simulink model "ES249B_MotAgCorrln"  (R2013b)
settings: Solver=FixedStepDiscrete  SolverMode=SingleTasking  StartTime=0.0  StopTime=1  FixedStep=0.002  RelTol=1e-3
values from neighbouring files (symbols this model uses):
  FLTINJ_MOTAGCORRLN_MOTAGIDPTSIG = DataDict.Constant    [ES249B_MotAgCorrln_DataDict.m]
  HALFREV_MOTREV_U0P16 = DataDict.Constant    [ES249B_MotAgCorrln_DataDict.m]
  MOTAGACORRLNST_CNT_U08 = DataDict.Constant    [ES249B_MotAgCorrln_DataDict.m]
  MotAgAMotAgBCorrln = DataDict.NTC    [ES249B_MotAgCorrln_DataDict.m]
  MOTAGBCORRLNST_CNT_U08 = DataDict.Constant    [ES249B_MotAgCorrln_DataDict.m]
  MOTAGCORRLNERRTHD_MOTREVELEC_U0P16 = DataDict.Constant    [ES249B_MotAgCorrln_DataDict.m]
  MOTAGCORRLNNTCFAILSTEP_CNT_U16 = DataDict.Constant    [ES249B_MotAgCorrln_DataDict.m]
  MOTAGCORRLNNTCPASSSTEP_CNT_U16 = DataDict.Constant    [ES249B_MotAgCorrln_DataDict.m]
  MOTAGMAXSTALLCNTR_CNT_U08 = DataDict.Constant    [ES249B_MotAgCorrln_DataDict.m]
  MotAgMeclCorrlnSt = DataDict.OpSignal    [ES249B_MotAgCorrln_DataDict.m]
  MotAgMeclIdptSig = DataDict.OpSignal    [ES249B_MotAgCorrln_DataDict.m]
  SysGlbPrmMotPoleCnt = DataDict.ImprtdCal    [ES249B_MotAgCorrln_DataDict.m]
undefined symbols (not defined in the file or in its folder): NtcSts1, sigbuilder_block, SigQlfr1
libraries: simulink x5
(part 2 of 2)

== system ES249B_MotAgCorrln/MotAgCorrln/MotAgCorrlnPer1/MtrAgB SigAvlCheck ==
  note: Example of PIM declaration for StallCnt State Variable
      |
      | SnsrShoNameSens0StallCntPrev = DataDict.PIM;
      | SnsrShoNameSens0StallCntPrev.LongName = 'SnsrShoNameSens0RollgCntPrev';
      | SnsrShoNameSens0StallCntPrev.Description = 'SnsrShoNameSens0RollgCntPrev';
      | SnsrShoNameSens0StallCntPrev.DocUnits = 'Cnt';
      | SnsrShoNameSens0StallCntPrev.EngDT = dt.u08;
      | SnsrShoNameSens0StallCntPrev.EngInit = 0;
      | SnsrShoNameSens0StallCntPrev.EngMin = 0;
      | SnsrShoNameSens0StallCntPrev.EngMax = 255;
      |
      |
      | *********  Need different state variable for each instance of this  subsystem ********
  note: Example of PIM declaration for RollgCnt State Variable
      |
      | SnsrShoNameSens0RollgCntPrev = DataDict.PIM;
      | SnsrShoNameSens0RollgCntPrev.LongName = 'SnsrShoNameSens0RollgCntPrev';
      | SnsrShoNameSens0RollgCntPrev.Description = 'SnsrShoNameSens0RollgCntPrev';
      | SnsrShoNameSens0RollgCntPrev.DocUnits = 'Cnt';
      | SnsrShoNameSens0RollgCntPrev.EngDT = dt.u08;
      | SnsrShoNameSens0RollgCntPrev.EngInit = 0;
      | SnsrShoNameSens0RollgCntPrev.EngMin = 0;
      | SnsrShoNameSens0RollgCntPrev.EngMax = 255;
      |
      |
      | *********  Need different state variable for each instance of this  subsystem ********
  SigRollgCnt : Inport  OutDataTypeStr=uint8
  SigQlfr : Inport  Port=2  OutDataTypeStr=uint8
  kMaxStallCnt : Inport  Port=3  OutDataTypeStr=uint8
  Copyright1 : Subsystem  Description=|  RequirementInfo={} %GIDa_9de21268_1023_46e5_9fbe_013ff02661ff  mask(Copyright Information){none=on}
      | Copyright info block.                                               
      |                                                                     
      | Place copyright information at the top of every subsystem in design.
      mask prompts: none "No parameters"
      mask help: Place copyright information at the top of every subsystem in design.
      mask Display:
      | NxtrConf = 'Nexteer Confidential';
      | 
      | sys = bdroot; %handle for the current model ("system")
      | first = get_param(sys,'Created');
      | if(isempty(first))
      |     first = datestr(now,'yyyy');
      | else
      |     first = first(end-3:end);  %year is last four digits
      | end
      | 
      | last = get_param(sys,'LastModifiedDate');
      | if isempty(last)
      |     last = datestr(now,'yyyy');
      | else
      |     last = last(end-3:end);
      | end
      | 
      | if strcmp(first,last)
      |     fprintf('%s\nCopyright  %s Nexteer',NxtrConf,first);
      | else
      |     fprintf('%s\n%s%s-%s Nexteer',NxtrConf,char(169),first,last);
      | end
  CorrSigAvlChkRev1 : Stateflow chart  TreatAsAtomicUnit=on
  Unit Delay : UnitDelay  SampleTime=-1  StateName=MotAgCorrlnMotAgBRollgCntPrev  StateMustResolveToSignalObject=on
      settings: AttributesFormatString=|
      | State Variable:
      | %<StateName>
  Unit Delay1 : UnitDelay  SampleTime=-1  StateName=MotAgCorrlnMotAgBStallCntPrev  StateMustResolveToSignalObject=on
      settings: AttributesFormatString=|
      | State Variable:
      | %<StateName>
  SigAvl : Outport
  wires:
  SigRollgCnt/1 -> Unit Delay/1, CorrSigAvlChkRev1/1(SigRollgCnt)  "SigRollgCnt"
  SigQlfr/1 -> CorrSigAvlChkRev1/2(SigQlfr)  "SigQlfr"
  kMaxStallCnt/1 -> CorrSigAvlChkRev1/3(kMaxStallCnt)  "kMaxStallCnt"
  Unit Delay/1 -> CorrSigAvlChkRev1/4(LstRollgCnt)
  CorrSigAvlChkRev1/2(StallCntOutp) -> Unit Delay1/1
  Unit Delay1/1 -> CorrSigAvlChkRev1/5(LstStallCnt)
  CorrSigAvlChkRev1/1(SigAvl) -> SigAvl/1

== system ES249B_MotAgCorrln/MotAgCorrln/MotAgCorrlnInit1/Compute Error Threshold/Copyright1 ==

== system ES249B_MotAgCorrln/MotAgCorrln/MotAgCorrlnPer1/Build Correlation Status/Copyright1 ==

== system ES249B_MotAgCorrln/MotAgCorrln/MotAgCorrlnPer1/DetermineIndSignals/Fail Action  ==
  Action Port : ActionPort  ActionType=else
  Constant : Constant  Value=0  OutDataTypeStr=uint8
      settings: AttributesFormatString=%<OutDataTypeStr>
  Copyright1 : Subsystem  Description=|  mask(Copyright Information){none=on}
      | Copyright info block.                                               
      |                                                                     
      | Place copyright information at the top of every subsystem in design.
      mask prompts: none "No parameters"
      mask help: Place copyright information at the top of every subsystem in design.
      mask Display:
      | NxtrConf = 'Nexteer Confidential';
      | 
      | sys = bdroot; %handle for the current model ("system")
      | first = get_param(sys,'Created');
      | if(isempty(first))
      |     first = datestr(now,'yyyy');
      | else
      |     first = first(end-3:end);  %year is last four digits
      | end
      | 
      | last = get_param(sys,'LastModifiedDate');
      | if isempty(last)
      |     last = datestr(now,'yyyy');
      | else
      |     last = last(end-3:end);
      | end
      | 
      | if strcmp(first,last)
      |     fprintf('%s\nCopyright  %s Nexteer',NxtrConf,first);
      | else
      |     fprintf('%s\n%s%s-%s Nexteer',NxtrConf,char(169),first,last);
      | end
  MotAgMeclIdptSig : Outport  OutDataTypeStr=uint8
  wires:
  Constant/1 -> MotAgMeclIdptSig/1

== system ES249B_MotAgCorrln/MotAgCorrln/MotAgCorrlnPer1/DetermineIndSignals/Pass Action  ==
  Action Port : ActionPort  ActionType=then
  Constant : Constant  Value=MotAgMeclIdptSig.EngMax  OutDataTypeStr=uint8
      settings: AttributesFormatString=%<OutDataTypeStr>
  Copyright1 : Subsystem  Description=|  mask(Copyright Information){none=on}
      | Copyright info block.                                               
      |                                                                     
      | Place copyright information at the top of every subsystem in design.
      mask prompts: none "No parameters"
      mask help: Place copyright information at the top of every subsystem in design.
      mask Display:
      | NxtrConf = 'Nexteer Confidential';
      | 
      | sys = bdroot; %handle for the current model ("system")
      | first = get_param(sys,'Created');
      | if(isempty(first))
      |     first = datestr(now,'yyyy');
      | else
      |     first = first(end-3:end);  %year is last four digits
      | end
      | 
      | last = get_param(sys,'LastModifiedDate');
      | if isempty(last)
      |     last = datestr(now,'yyyy');
      | else
      |     last = last(end-3:end);
      | end
      | 
      | if strcmp(first,last)
      |     fprintf('%s\nCopyright  %s Nexteer',NxtrConf,first);
      | else
      |     fprintf('%s\n%s%s-%s Nexteer',NxtrConf,char(169),first,last);
      | end
  MotAgMeclIdptSig : Outport
  wires:
  Constant/1 -> MotAgMeclIdptSig/1

== system ES249B_MotAgCorrln/MotAgCorrln/MotAgCorrlnPer1/FltInj_u08 /Copyright1 ==

== system ES249B_MotAgCorrln/MotAgCorrln/MotAgCorrlnPer1/GetNtcQlfrSts 0x080 /CopyRight2 ==

== system ES249B_MotAgCorrln/MotAgCorrln/MotAgCorrlnPer1/MotAgA vs MotAgB/Copyright1 ==

== system ES249B_MotAgCorrln/MotAgCorrln/MotAgCorrlnPer1/MotAgA vs MotAgB/Fails the test ==
  Action Port : ActionPort  ActionType=else
  Copyright1 : Subsystem  Description=|  mask(Copyright Information){none=on}
      | Copyright info block.                                               
      |                                                                     
      | Place copyright information at the top of every subsystem in design.
      mask prompts: none "No parameters"
      mask help: Place copyright information at the top of every subsystem in design.
      mask Display:
      | NxtrConf = 'Nexteer Confidential';
      | 
      | sys = bdroot; %handle for the current model ("system")
      | first = get_param(sys,'Created');
      | if(isempty(first))
      |     first = datestr(now,'yyyy');
      | else
      |     first = first(end-3:end);  %year is last four digits
      | end
      | 
      | last = get_param(sys,'LastModifiedDate');
      | if isempty(last)
      |     last = datestr(now,'yyyy');
      | else
      |     last = last(end-3:end);
      | end
      | 
      | if strcmp(first,last)
      |     fprintf('%s\nCopyright  %s Nexteer',NxtrConf,first);
      | else
      |     fprintf('%s\n%s%s-%s Nexteer',NxtrConf,char(169),first,last);
      | end
  MOTAGCORRLNNTCFAILSTEP_CNT_U16 : Constant  Value=MOTAGCORRLNNTCFAILSTEP_CNT_U16
  Parameter Byte : Constant  OutDataTypeStr=uint8
  Status Type : Constant  Value=NtcSts1.NTCSTS_PREFAILD
  NtcInfo : Outport  InitialOutput=1
  NtcSts : Outport  Port=2  InitialOutput=NtcSts1.NTCSTS_PREFAILD
  DebStep : Outport  Port=3  InitialOutput=MOTAGCORRLNNTCFAILSTEP_CNT_U16
  wires:
  MOTAGCORRLNNTCFAILSTEP_CNT_U16/1 -> DebStep/1
  Status Type/1 -> NtcSts/1
  Parameter Byte/1 -> NtcInfo/1

== system ES249B_MotAgCorrln/MotAgCorrln/MotAgCorrlnPer1/MotAgA vs MotAgB/Passes the test ==
  Action Port : ActionPort  ActionType=then
  Copyright1 : Subsystem  Description=|  mask(Copyright Information){none=on}
      | Copyright info block.                                               
      |                                                                     
      | Place copyright information at the top of every subsystem in design.
      mask prompts: none "No parameters"
      mask help: Place copyright information at the top of every subsystem in design.
      mask Display:
      | NxtrConf = 'Nexteer Confidential';
      | 
      | sys = bdroot; %handle for the current model ("system")
      | first = get_param(sys,'Created');
      | if(isempty(first))
      |     first = datestr(now,'yyyy');
      | else
      |     first = first(end-3:end);  %year is last four digits
      | end
      | 
      | last = get_param(sys,'LastModifiedDate');
      | if isempty(last)
      |     last = datestr(now,'yyyy');
      | else
      |     last = last(end-3:end);
      | end
      | 
      | if strcmp(first,last)
      |     fprintf('%s\nCopyright  %s Nexteer',NxtrConf,first);
      | else
      |     fprintf('%s\n%s%s-%s Nexteer',NxtrConf,char(169),first,last);
      | end
  MOTAGCORRLNNTCPASSSTEP_CNT_U16 : Constant  Value=MOTAGCORRLNNTCPASSSTEP_CNT_U16
  Parameter Byte Data1 : Constant  Value=0  OutDataTypeStr=uint8
  Status Type : Constant  Value=NtcSts1.NTCSTS_PREPASSD
  NtcInfo : Outport  InitialOutput=0
  NtcSts : Outport  Port=2  InitialOutput=NtcSts1.NTCSTS_PREPASSD
  DebStep : Outport  Port=3  InitialOutput=MOTAGCORRLNNTCPASSSTEP_CNT_U16
  wires:
  MOTAGCORRLNNTCPASSSTEP_CNT_U16/1 -> DebStep/1
  Status Type/1 -> NtcSts/1
  Parameter Byte Data1/1 -> NtcInfo/1

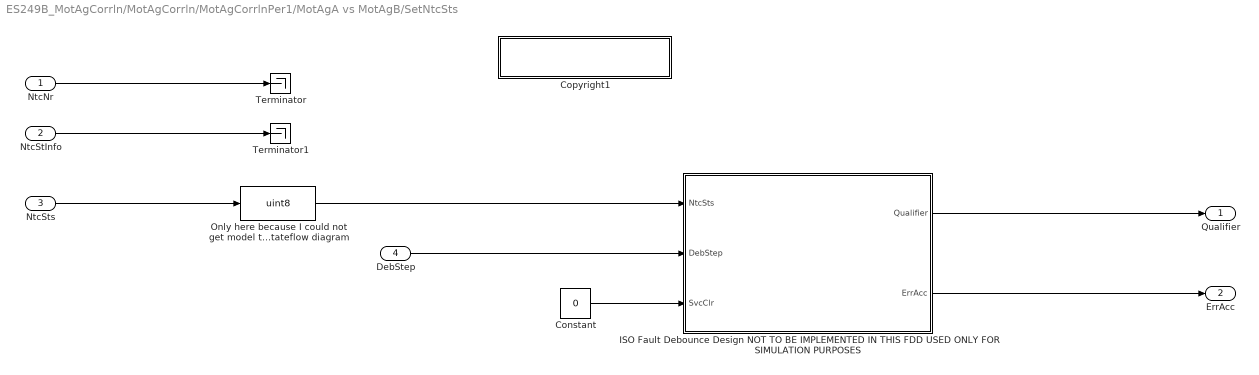
== system ES249B_MotAgCorrln/MotAgCorrln/MotAgCorrlnPer1/MotAgA vs MotAgB/SetNtcSts ==
  NtcNr : Inport
  NtcStInfo : Inport  Port=2
  NtcSts : Inport  Port=3  OutDataTypeStr=Enum: NtcSts1
  DebStep : Inport  Port=4  OutDataTypeStr=uint16
  Constant : Constant  Value=0
  Copyright1 : Subsystem  Description=|  mask(Copyright Information){none=on}
      | Copyright info block.                                               
      |                                                                     
      | Place copyright information at the top of every subsystem in design.
      mask prompts: none "No parameters"
      mask help: Place copyright information at the top of every subsystem in design.
      mask Display:
      | NxtrConf = 'Nexteer Confidential';
      | 
      | sys = bdroot; %handle for the current model ("system")
      | first = get_param(sys,'Created');
      | if(isempty(first))
      |     first = datestr(now,'yyyy');
      | else
      |     first = first(end-3:end);  %year is last four digits
      | end
      | 
      | last = get_param(sys,'LastModifiedDate');
      | if isempty(last)
      |     last = datestr(now,'yyyy');
      | else
      |     last = last(end-3:end);
      | end
      | 
      | if strcmp(first,last)
      |     fprintf('%s\nCopyright  %s Nexteer',NxtrConf,first);
      | else
      |     fprintf('%s\n%s%s-%s Nexteer',NxtrConf,char(169),first,last);
      | end
  ISO Fault Debounce Design NOT TO BE IMPLEMENTED IN THIS FDD USED ONLY FOR SIMULATION PURPOSES : Stateflow chart  TreatAsAtomicUnit=on
  Only here because I could not get model to run with enumerations in the stateflow diagram : DataTypeConversion  OutDataTypeStr=uint8
  Terminator : Terminator
  Terminator1 : Terminator
  Qualifier : Outport
  ErrAcc : Outport  Port=2
  wires:
  Only here because I could not get model to run with enumerations in the stateflow diagram/1 -> ISO Fault Debounce Design NOT TO BE IMPLEMENTED IN THIS FDD USED ONLY FOR SIMULATION PURPOSES/1(NtcSts)
  ISO Fault Debounce Design NOT TO BE IMPLEMENTED IN THIS FDD USED ONLY FOR SIMULATION PURPOSES/2(ErrAcc) -> ErrAcc/1
  Constant/1 -> ISO Fault Debounce Design NOT TO BE IMPLEMENTED IN THIS FDD USED ONLY FOR SIMULATION PURPOSES/3(SvcClr)
  ISO Fault Debounce Design NOT TO BE IMPLEMENTED IN THIS FDD USED ONLY FOR SIMULATION PURPOSES/1(Qualifier) -> Qualifier/1
  DebStep/1 -> ISO Fault Debounce Design NOT TO BE IMPLEMENTED IN THIS FDD USED ONLY FOR SIMULATION PURPOSES/2(DebStep)
  NtcSts/1 -> Only here because I could not get model to run with enumerations in the stateflow diagram/1
  NtcNr/1 -> Terminator/1
  NtcStInfo/1 -> Terminator1/1

== system ES249B_MotAgCorrln/MotAgCorrln/MotAgCorrlnPer1/MtrAgA SigAvlCheck/Copyright1 ==

== system ES249B_MotAgCorrln/MotAgCorrln/MotAgCorrlnPer1/MtrAgB SigAvlCheck/Copyright1 ==

== system ES249B_MotAgCorrln/MotAgCorrln/MotAgCorrlnPer1/DetermineIndSignals/Fail Action /Copyright1 ==

== system ES249B_MotAgCorrln/MotAgCorrln/MotAgCorrlnPer1/DetermineIndSignals/Pass Action /Copyright1 ==

== system ES249B_MotAgCorrln/MotAgCorrln/MotAgCorrlnPer1/MotAgA vs MotAgB/Fails the test/Copyright1 ==

== system ES249B_MotAgCorrln/MotAgCorrln/MotAgCorrlnPer1/MotAgA vs MotAgB/Passes the test/Copyright1 ==

== system ES249B_MotAgCorrln/MotAgCorrln/MotAgCorrlnPer1/MotAgA vs MotAgB/SetNtcSts/Copyright1 ==

== stateflow chart ES249B_MotAgCorrln/MotAgCorrln/MotAgCorrlnPer1/MotAgA vs MotAgB/SetNtcSts/ISO Fault Debounce Design NOT TO BE IMPLEMENTED IN THIS FDD USED ONLY FOR SIMULATION PURPOSES ==
  note: NTCSTS_PASSD           (0)
      | NTCSTS_FAILD             (1)
      | NTCSTS_PREPASSD   (2)
      | NTCSTS_PREFAILD     (3)
      |
      | SIGQLFR_NORES        (0)
      | SIGQLFR_PASSD         (1)
      | SIGQLFR_FAILD           (2)
  note: Nstep Loop
  note: Pstep Loop
  note: 
  (default) -> (junction 89)
  (junction 89) -> (junction 95) [order 1] : [NtcSts == 3]
  (junction 89) -> (junction 93) [order 2] : [ NtcSts == 2]
  (junction 93) -> (junction 230) [order 2] : {
      | ErrAcc = ErrAcc - DebStep;
      | }
  (junction 95) -> (junction 213) [order 1] : [ErrAcc <=0]
      | {
      | ErrAcc = DebStep;
      | }
  (junction 95) -> (junction 103) [order 2]
  (junction 89) -> (junction 221) [order 3] : [(NtcSts == 0) | ...
      | (NtcSts == 1)]
  (junction 93) -> (junction 123) [order 1] : [(ErrAcc - DebStep) <= -32768]
      | {
      | ErrAcc = -32768;
      | Qualifier = 1;
      | }
  (junction 230) -> (junction 231)
  (junction 213) -> (junction 216)
  (junction 103) -> (junction 216) [order 2] : {
      | ErrAcc = ErrAcc + DebStep;
      | }
  (junction 221) -> (junction 222) [order 2] : [NtcSts == 0]
      | {
      | ErrAcc = -32768;
      | Qualifier=1;
      | }
  (junction 216) -> (junction 214)
  (junction 103) -> (junction 220) [order 1] : [(ErrAcc + DebStep) >=32767]
      | {
      | ErrAcc = 32767;
      | Qualifier =2;
      | }
  (junction 221) -> (junction 212) [order 1] : [NtcSts == 1]
      | {
      | ErrAcc = 32767;
      | Qualifier =2;
      |  }
  (junction 222) -> (junction 225)
  (junction 225) -> (junction 212)
  (junction 212) -> (junction 141)
  (junction 214) -> (junction 220)
  (junction 220) -> (junction 141)
  (junction 123) -> (junction 141)
  (junction 231) -> (junction 123)
  (junction 141) -> (junction 159)
  (junction 159) -> (junction 235) [order 2]
  (junction 235) -> (junction 236)
  (junction 159) -> (junction 234) [order 1] : [SvcClr ==1]
      | {
      | ErrAcc = 0;
      | Qualifier =0;
      | }
  (junction 236) -> (junction 234)
  data: NtcSts input uint8; Qualifier output uint8; DebStep input uint16; ErrAcc output int16; SvcClr input

== stateflow chart ES249B_MotAgCorrln/MotAgCorrln/MotAgCorrlnPer1/MtrAgB SigAvlCheck/CorrSigAvlChkRev1 ==
  note: SigAvl
      | False = 0
      | Pass = 1
  note: SigQlfr
      | 0 = No Result
      | 1 = Pass
      | 2 = Fail
  (default) -> (junction 2)
  (junction 2) -> (junction 4) [order 1] : [SigRollgCnt ==LstRollgCnt]
  (junction 4) -> (junction 7) [order 2] : {
      | StallCntOutp = LstStallCnt +1;
      | }
  (junction 2) -> (junction 3) [order 2]
  (junction 4) -> (junction 7) [order 1] : [LstStallCnt == 255]
      | {
      | StallCntOutp = 255;
      | }
  (junction 3) -> (junction 7) : {
      | StallCntOutp = 0;
      | }
  (junction 7) -> (junction 10)
  (junction 10) -> (junction 12) [order 1] : [StallCntOutp >=kMaxStallCnt]
  (junction 10) -> (junction 14) [order 2]
  (junction 12) -> (junction 17)
  (junction 14) -> (junction 17) [order 2]
  (junction 14) -> (junction 16) [order 1] : [SigQlfr<2]
  (junction 17) -> (junction 29) : {
      | SigAvl =0;
      | }
  (junction 16) -> (junction 29) : {
      | SigAvl = 1;
      | }
  data: SigRollgCnt input; SigQlfr input; kMaxStallCnt input; SigAvl output boolean; LstRollgCnt input uint8; LstStallCnt input uint8; StallCntOutp output uint8

== stateflow chart ES249B_MotAgCorrln/MotAgCorrln/MotAgCorrlnPer1/MtrAgA SigAvlCheck/CorrSigAvlChkRev1 ==
  note: SigAvl
      | False = 0
      | Pass = 1
  note: SigQlfr
      | 0 = No Result
      | 1 = Pass
      | 2 = Fail
  (default) -> (junction 2)
  (junction 2) -> (junction 4) [order 1] : [SigRollgCnt ==LstRollgCnt]
  (junction 4) -> (junction 7) [order 2] : {
      | StallCntOutp = LstStallCnt +1;
      | }
  (junction 2) -> (junction 3) [order 2]
  (junction 4) -> (junction 7) [order 1] : [LstStallCnt == 255]
      | {
      | StallCntOutp = 255;
      | }
  (junction 3) -> (junction 7) : {
      | StallCntOutp = 0;
      | }
  (junction 7) -> (junction 10)
  (junction 10) -> (junction 12) [order 1] : [StallCntOutp >=kMaxStallCnt]
  (junction 10) -> (junction 14) [order 2]
  (junction 12) -> (junction 17)
  (junction 14) -> (junction 17) [order 2]
  (junction 14) -> (junction 16) [order 1] : [SigQlfr<2]
  (junction 17) -> (junction 29) : {
      | SigAvl =0;
      | }
  (junction 16) -> (junction 29) : {
      | SigAvl = 1;
      | }
  data: SigRollgCnt input; SigQlfr input; kMaxStallCnt input; SigAvl output boolean; LstRollgCnt input uint8; LstStallCnt input uint8; StallCntOutp output uint8
